simulink model "fullStateFeadback"  (R2024a)
settings: Solver=VariableStepAuto  StartTime=0.0  StopTime=t_sim  RelTol=1e-3
values from neighbouring files (symbols this model uses):
  C = [0 1 1]    [SISO.m]    (also in invertedPendulum.m = [-1 0 0 0; invertedPendulumSys.m = [-1 0 0 0)
  K = acker(A_aug, B_aug, l_des)    [SISO.m]    (also in invertedPendulum.m = acker(A,B,des); invertedPendulumSys.m = acker(A,B,des))
libraries: cstblocks x1
settings Model: Creator=lorenzo  LastModifiedBy=lorenzo

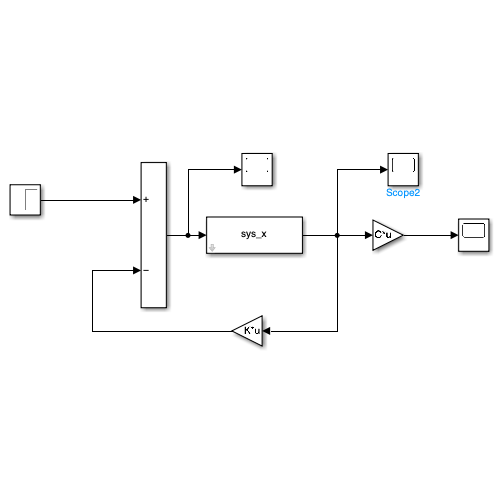
[thumbnail: Simulink's stored preview of the top-level diagram]
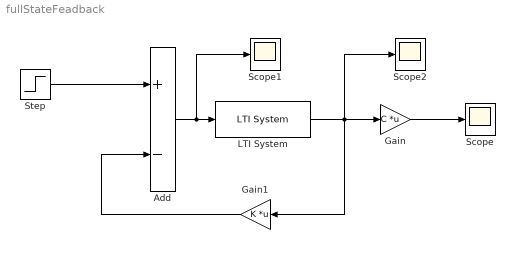
== system fullStateFeadback ==
  Add : Sum  Inputs=+-
  Gain : Gain  Gain=C  Multiplication=Matrix(K*u)
  Gain1 : Gain  Gain=K  Multiplication=Matrix(K*u)
  LTI System : cstblocks/LTI System  sys=sys_x  IC=x0  PadeOrder=0
  Scope : Scope
  Scope1 : Scope
  Scope2 : Scope
  Step : Step  SampleTime=0
  wires:
  LTI System/1 -> Scope2/1, Gain/1, Gain1/1
  Gain1/1 -> Add/2
  Step/1 -> Add/1
  Gain/1 -> Scope/1
  Add/1 -> Scope1/1, LTI System/1
